simulink model "analyse_3310"  (R2017b)
settings: Solver=ode5  StartTime=0.0  StopTime=1  FixedStep=1e-3  RelTol=1e-3
libraries: simulink x2
settings Model: Creator=dqviet  LastModifiedBy=dqviet

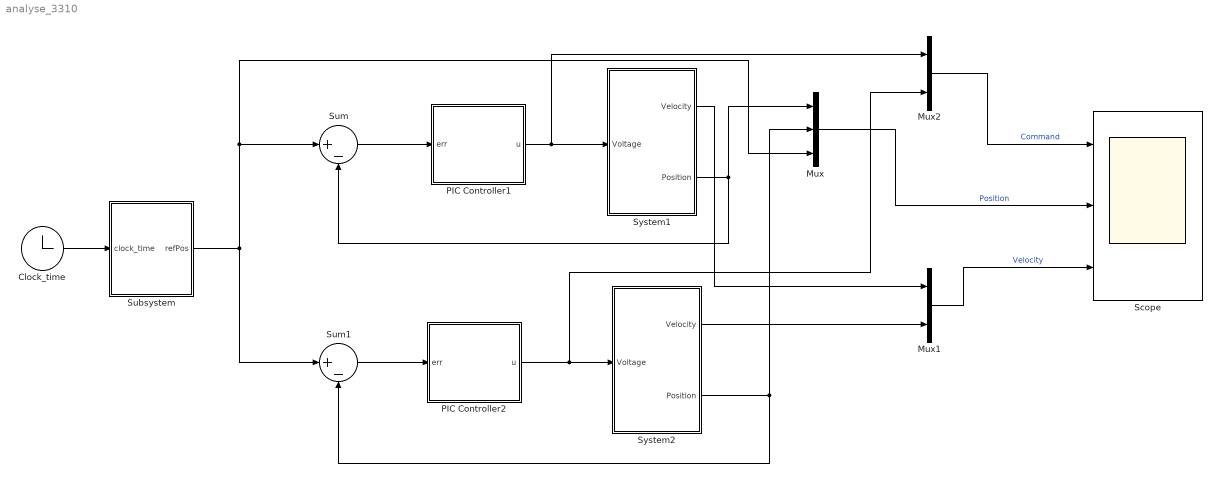
== system analyse_3310 ==
  Clock_time : Clock
  Mux : Mux  Inputs=3
  Mux1 : Mux  Inputs=2
  Mux2 : Mux  Inputs=2
  PIC Controller1 : Subsystem
  PIC Controller2 : Subsystem
  Scope : Scope  NumInputPorts=3
  Subsystem : Subsystem
  Sum : Sum  Inputs=|+-
  Sum1 : Sum  Inputs=|+-
  "System1 " : Subsystem
  System2 : Subsystem
  wires:
  Clock_time/1 -> Subsystem/1(clock_time)
  "System1 "/2(Position) -> Mux/1, Sum/2
  Sum/1 -> PIC Controller1/1(err)
  PIC Controller1/1(u) -> Mux2/1, "System1 "/1(Voltage)
  PIC Controller2/1(u) -> Mux2/2, System2/1(Voltage)
  Sum1/1 -> PIC Controller2/1(err)
  System2/2(Position) -> Mux/2, Sum1/2
  Subsystem/1(refPos) -> Mux/3, Sum/1, Sum1/1
  Mux/1 -> Scope/2  "Position"
  "System1 "/1(Velocity) -> Mux1/1
  System2/1(Velocity) -> Mux1/2
  Mux1/1 -> Scope/3  "Velocity"
  Mux2/1 -> Scope/1  "Command"

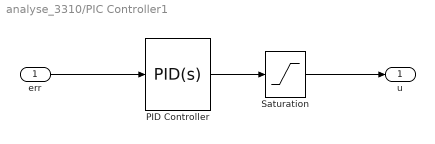
== system analyse_3310/PIC Controller1 ==
  err : Inport
  PID Controller : simulink/Continuous/PID Controller  Controller=PID  TimeDomain=Continuous-time  SampleTime=-1  IntegratorMethod=Forward Euler  FilterMethod=Forward Euler  Form=Parallel  UseFilter=on  ControllerParametersSource=internal  P=1e+4  I=0  D=1e+2  N=100  InitialConditionSource=internal  InitialConditionForIntegrator=0  InitialConditionForFilter=0  ExternalReset=none  LimitOutput=off  UpperSaturationLimit=inf  LowerSaturationLimit=-inf  LinearizeAsGain=on  AntiWindupMode=none  Kb=1  TrackingMode=off  Kt=1  PParamMin=[]  PParamMax=[]  IParamMin=[]  IParamMax=[]  DParamMin=[]  DParamMax=[]  NParamMin=[]  NParamMax=[]  KbParamMin=[]  KbParamMax=[]  KtParamMin=[]  KtParamMax=[]  POutMin=[]  POutMax=[]  IOutMin=[]  IOutMax=[]  DOutMin=[]  DOutMax=[]  NOutMin=[]  NOutMax=[]  KbOutMin=[]  KbOutMax=[]  KtOutMin=[]  KtOutMax=[]  IntegratorOutMin=[]  IntegratorOutMax=[]  FilterOutMin=[]  FilterOutMax=[]  SumOutMin=[]  SumOutMax=[]  SumI1OutMin=[]  SumI1OutMax=[]  SumI2OutMin=[]  SumI2OutMax=[]  SumI3OutMin=[]  SumI3OutMax=[]  SumDOutMin=[]  SumDOutMax=[]  SaturationOutMin=[]  SaturationOutMax=[]  IntegratorContinuousStateAttributes=''  IntegratorStateMustResolveToSignalObject=off  IntegratorRTWStateStorageClass=Auto  FilterContinuousStateAttributes=''  FilterStateMustResolveToSignalObject=off  FilterRTWStateStorageClass=Auto  DifferentiatorICPrevScaledInput=0  DifferentiatorOutMin=[]  DifferentiatorOutMax=[]  InitialConditionSetting=State (most efficient)  FilterDiffOutCoefMin=[]  FilterDiffOutCoefMax=[]  SumDenOutMin=[]  SumDenOutMax=[]  SumNumOutMin=[]  SumNumOutMax=[]  ReciprocalOutMin=[]  ReciprocalOutMax=[]  DivideOutMin=[]  DivideOutMax=[]  TunerSelectOption=Transfer Function Based (PID Tuner App)
  Saturation : Saturate  UpperLimit=15  LowerLimit=-15
  u : Outport
  wires:
  Saturation/1 -> u/1
  PID Controller/1 -> Saturation/1
  err/1 -> PID Controller/1

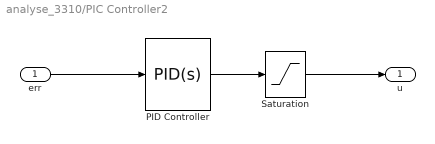
== system analyse_3310/PIC Controller2 ==
  err : Inport
  PID Controller : simulink/Continuous/PID Controller  Controller=PID  TimeDomain=Continuous-time  SampleTime=-1  IntegratorMethod=Forward Euler  FilterMethod=Forward Euler  Form=Parallel  UseFilter=on  ControllerParametersSource=internal  P=1e+3  I=0  D=1e+2  N=100  InitialConditionSource=internal  InitialConditionForIntegrator=0  InitialConditionForFilter=0  ExternalReset=none  LimitOutput=off  UpperSaturationLimit=inf  LowerSaturationLimit=-inf  LinearizeAsGain=on  AntiWindupMode=none  Kb=1  TrackingMode=off  Kt=1  PParamMin=[]  PParamMax=[]  IParamMin=[]  IParamMax=[]  DParamMin=[]  DParamMax=[]  NParamMin=[]  NParamMax=[]  KbParamMin=[]  KbParamMax=[]  KtParamMin=[]  KtParamMax=[]  POutMin=[]  POutMax=[]  IOutMin=[]  IOutMax=[]  DOutMin=[]  DOutMax=[]  NOutMin=[]  NOutMax=[]  KbOutMin=[]  KbOutMax=[]  KtOutMin=[]  KtOutMax=[]  IntegratorOutMin=[]  IntegratorOutMax=[]  FilterOutMin=[]  FilterOutMax=[]  SumOutMin=[]  SumOutMax=[]  SumI1OutMin=[]  SumI1OutMax=[]  SumI2OutMin=[]  SumI2OutMax=[]  SumI3OutMin=[]  SumI3OutMax=[]  SumDOutMin=[]  SumDOutMax=[]  SaturationOutMin=[]  SaturationOutMax=[]  IntegratorContinuousStateAttributes=''  IntegratorStateMustResolveToSignalObject=off  IntegratorRTWStateStorageClass=Auto  FilterContinuousStateAttributes=''  FilterStateMustResolveToSignalObject=off  FilterRTWStateStorageClass=Auto  DifferentiatorICPrevScaledInput=0  DifferentiatorOutMin=[]  DifferentiatorOutMax=[]  InitialConditionSetting=State (most efficient)  FilterDiffOutCoefMin=[]  FilterDiffOutCoefMax=[]  SumDenOutMin=[]  SumDenOutMax=[]  SumNumOutMin=[]  SumNumOutMax=[]  ReciprocalOutMin=[]  ReciprocalOutMax=[]  DivideOutMin=[]  DivideOutMax=[]  TunerSelectOption=Transfer Function Based (PID Tuner App)
  Saturation : Saturate  UpperLimit=15  LowerLimit=-15
  u : Outport
  wires:
  Saturation/1 -> u/1
  PID Controller/1 -> Saturation/1
  err/1 -> PID Controller/1

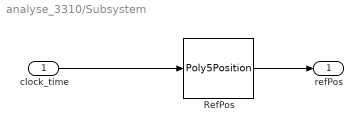
== system analyse_3310/Subsystem ==
  clock_time : Inport
  RefPos : MATLABFcn  MATLABFcn=Poly5Position
  refPos : Outport
  wires:
  RefPos/1 -> refPos/1
  clock_time/1 -> RefPos/1

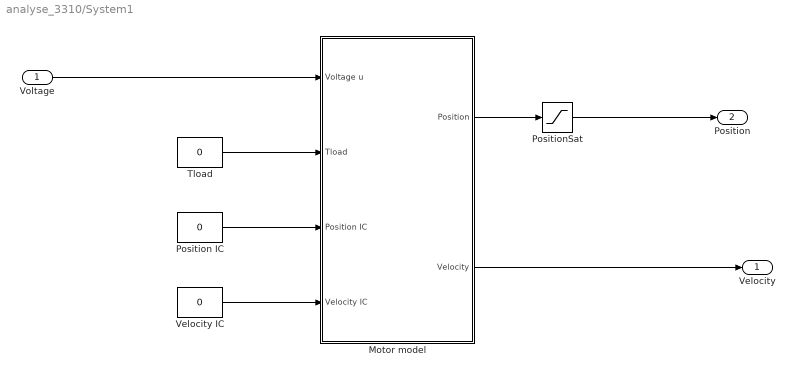
== system analyse_3310/System1  ==
  Voltage : Inport
  Motor model : Subsystem
  Position IC : Constant  Value=0
  PositionSat : Saturate
  Tload : Constant  Value=0
  Velocity IC : Constant  Value=0
  Velocity : Outport
  Position : Outport  Port=2
  wires:
  Motor model/2(Velocity) -> Velocity/1
  Voltage/1 -> Motor model/1(Voltage u)
  Tload/1 -> Motor model/2(Tload)
  Velocity IC/1 -> Motor model/4(Velocity IC)
  Position IC/1 -> Motor model/3(Position IC)
  Motor model/1(Position) -> PositionSat/1
  PositionSat/1 -> Position/1

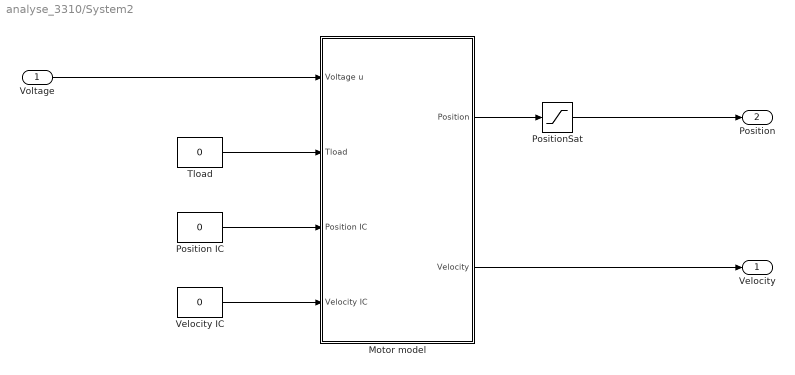
== system analyse_3310/System2 ==
  Voltage : Inport
  Motor model : Subsystem
  Position IC : Constant  Value=0
  PositionSat : Saturate
  Tload : Constant  Value=0
  Velocity IC : Constant  Value=0
  Velocity : Outport
  Position : Outport  Port=2
  wires:
  Motor model/2(Velocity) -> Velocity/1
  Voltage/1 -> Motor model/1(Voltage u)
  Tload/1 -> Motor model/2(Tload)
  Velocity IC/1 -> Motor model/4(Velocity IC)
  Position IC/1 -> Motor model/3(Position IC)
  Motor model/1(Position) -> PositionSat/1
  PositionSat/1 -> Position/1

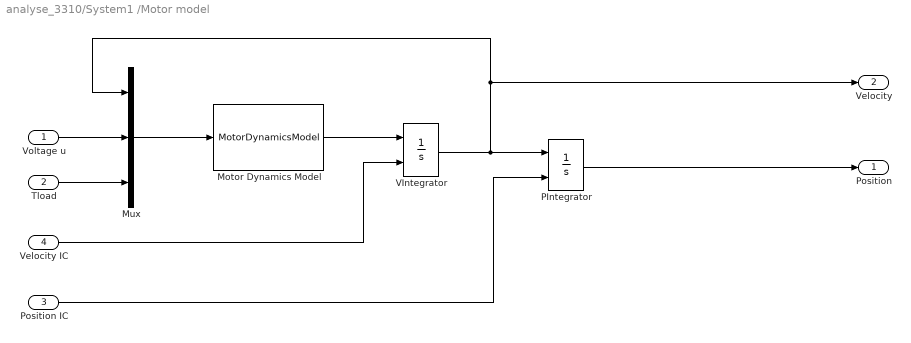
== system analyse_3310/System1 /Motor model ==
  Voltage u : Inport
  Tload : Inport  Port=2
  Position IC : Inport  Port=3
  Velocity IC : Inport  Port=4
  Motor Dynamics Model : MATLABFcn  MATLABFcn=MotorDynamicsModel
  Mux : Mux  Inputs=3
  PIntegrator : Integrator  InitialConditionSource=external
  "VIntegrator " : Integrator  InitialConditionSource=external
  Position : Outport
  Velocity : Outport  Port=2
  wires:
  "VIntegrator "/1 -> PIntegrator/1, Velocity/1, Mux/1
  Velocity IC/1 -> "VIntegrator "/2
  Position IC/1 -> PIntegrator/2
  Mux/1 -> Motor Dynamics Model/1
  Tload/1 -> Mux/3
  PIntegrator/1 -> Position/1
  Motor Dynamics Model/1 -> "VIntegrator "/1
  Voltage u/1 -> Mux/2

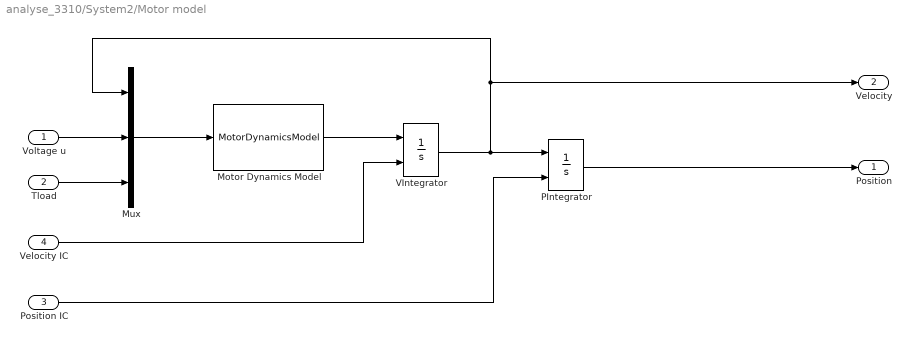
== system analyse_3310/System2/Motor model ==
  Voltage u : Inport
  Tload : Inport  Port=2
  Position IC : Inport  Port=3
  Velocity IC : Inport  Port=4
  Motor Dynamics Model : MATLABFcn  MATLABFcn=MotorDynamicsModel
  Mux : Mux  Inputs=3
  PIntegrator : Integrator  InitialConditionSource=external
  "VIntegrator " : Integrator  InitialConditionSource=external
  Position : Outport
  Velocity : Outport  Port=2
  wires:
  "VIntegrator "/1 -> PIntegrator/1, Velocity/1, Mux/1
  Velocity IC/1 -> "VIntegrator "/2
  Position IC/1 -> PIntegrator/2
  Mux/1 -> Motor Dynamics Model/1
  Tload/1 -> Mux/3
  PIntegrator/1 -> Position/1
  Motor Dynamics Model/1 -> "VIntegrator "/1
  Voltage u/1 -> Mux/2
